simulink model "C6_Fix"  (R2024b)
settings: Solver=daessc  StartTime=0.0  StopTime=10.0  RelTol=1e-3  EnableMultiTasking=on
values from neighbouring files (symbols this model uses):
  Ix1 = 0.000555447536833    [C6_workspace.mat]
  Ix2 = 0.000647276077146    [C6_workspace.mat]
  Ix3 = 0.000647276077146    [C6_workspace.mat]
  Ix4 = 0.00061268668168    [C6_workspace.mat]
  Iy1 = 0.000281297083333    [C6_workspace.mat]
  Iy2 = 0.000285516539583    [C6_workspace.mat]
  Iy3 = 0.000285516539583    [C6_workspace.mat]
  Iy4 = 0.000286923025    [C6_workspace.mat]
  Iz1 = 0.000673203786833    [C6_workspace.mat]
  Iz2 = 0.000766798670896    [C6_workspace.mat]
  Iz3 = 0.000766798670896    [C6_workspace.mat]
  Iz4 = 0.00073279805668    [C6_workspace.mat]
  m_1 = 2    [C6_workspace.mat]
  m_2 = 2.03    [C6_workspace.mat]
  m_3 = 2.03    [C6_workspace.mat]
  m_4 = 2.04    [C6_workspace.mat]
undefined symbols (not defined in the file or in its folder): X, Y, Z
libraries: sm_lib x115, nesl_utility x25, robotcorelib x3, stm32f4xxblockslib x1
(part 1 of 6)
settings Model: STM32="{\"PWMOutput\":{\"ID\":\"C6_Fix:466\"}}"  ExtModeTrigDuration=2  Creator=steph  LastModifiedBy=steph
settings OptimizationCC: DefaultParameterBehavior=Inlined  EnhancedBackFolding=on  PassReuseOutputArgsAs=Individual arguments  ZeroExternalMemoryAtStartup=off  ZeroInternalMemoryAtStartup=off  MaxStackSize=512  OptimizeBlockOrder=speed  DifferentSizesBufferReuse=on  OptimizationCustomize=off  EfficientTunableParamExpr=on
settings DebuggingCC: ParameterTunabilityLossMsg=error
settings HardwareCC: ProdBitPerPointer=32  ProdBitPerSizeT=32  ProdBitPerPtrDiffT=32  ProdLargestAtomicInteger=Long  ProdLargestAtomicFloat=Double  ProdWordSize=32  ProdLongLongMode=on  ProdHWDeviceType=ARM Compatible->ARM Cortex-M
settings SFSimCC: MATLABDynamicMemAlloc=off
settings RTWCC: Description=Embedded Coder  SystemTargetFile=ert.tlc  HardwareBoard=STM32F4xx Based  TemplateMakefile=ert_default_tmf  Toolchain=GNU Tools for ARM Embedded Processors  BuildConfiguration=Faster Runs
settings CodeAppCC: ForceParamTrailComments=on  IgnoreCustomStorageClasses=off  OperatorAnnotations=on  SimulinkDataObjDesc=on  SFDataObjDesc=on  InsertBlockDesc=on
settings ERTTargetCC: TargetLangStandard=C99 (ISO)  CodeReplacementLibrary=ARM Cortex-M  RemoveResetFunc=off  ExtModeTransport=3  ExtModeStaticAlloc=on  ExtModeStaticAllocSize=2048  ExtModeMexFile=ext_xcp  ExtModeIntrfLevel=Level2 - Open  ConvertIfToSwitch=off  SuppressUnreachableDefaultCases=off

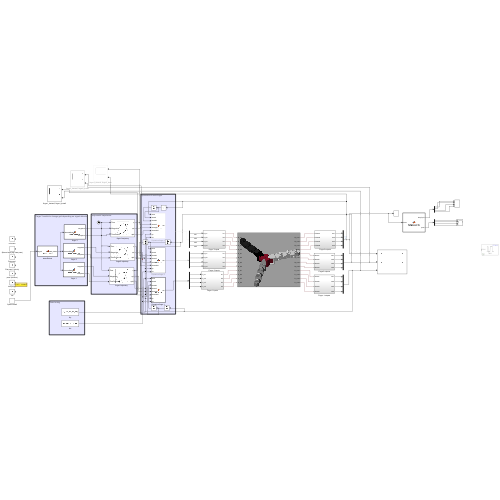
[thumbnail: Simulink's stored preview of the top-level diagram]
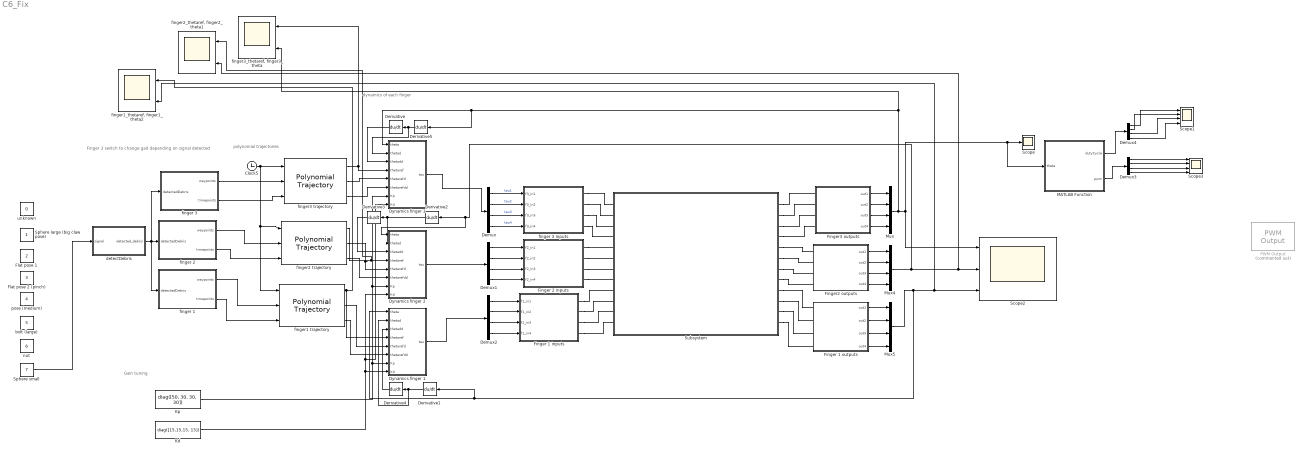
== system C6_Fix ==
  note: polynomial trajectories
  note: Gain tuning
  note: dynamics of each finger
  note: Finger 3 switch to change gait depending on signal detected
  Clock5 : Clock
  Demux{,1..4} (5 alike) : Demux
  Derivative{,1..5} (6 alike) : Derivative
  Dynamics finger 1 : MATLAB Function  TreatAsAtomicUnit=on
  Dynamics finger 2 : MATLAB Function  TreatAsAtomicUnit=on
  Dynamics finger 3 : MATLAB Function  TreatAsAtomicUnit=on
  Finger 1 inputs : Subsystem
  Finger 1 outputs : Subsystem
  Finger 2 inputs : Subsystem
  Finger2 outputs : Subsystem
  Finger3 outputs : Subsystem
  Flat pose 1 : Constant  Value=2
  Flat pose 2 (pinch) : Constant  Value=3
  Kd : Constant  Value=diag([15,15,15, 15])
  Kp : Constant  Value=diag([50, 30, 30, 30])
  MATLAB Function : MATLAB Function  TreatAsAtomicUnit=on
  Mux : Mux
  Mux4 : Mux
  Mux5 : Mux
  PWM Output : stm32f4xxblockslib/PWM Output  Commented=on  TimerModule=TIM1  DutycycleUnits=Percentage  EnableChannel1=on  EnableChannel2=off  EnableChannel3=off  EnableChannel4=off  EnableCounterInput=off  EnableMainOutputInput=off  EnableFrequencyInput=off  SetRCAfterCE=off  OutputDirection=off  OutputMainOutputEnableStatus=off  SampleTime=0.1  EnableSimPort=off  EnableUpdateEvent=off  EnableCaptureCompare1Event=off  EnableCaptureCompare2Event=off  EnableCaptureCompare3Event=off  EnableCaptureCompare4Event=off  EnableTriggerEvent=off  EnableBreakEvent=off  ProcessorFamily=STM32F4  hoistedMaskSrc=ECSoC/ECSimCodegen/PWM Output
  Scope : Scope
  Scope1 : Scope  NumInputPorts=4
  Scope2 : Scope  NumInputPorts=3
  Scope3 : Scope  NumInputPorts=4
  Sphere large (big claw pose) : Constant
  Sphere small : Constant  Value=7
  Subsystem : Subsystem
      mask Display: image('c6_fix.png');
  bolt (large) : Constant  Value=5
  detectDebris : MATLAB Function  TreatAsAtomicUnit=on
  finger 1 : MATLAB Function  TreatAsAtomicUnit=on
  finger 2 : MATLAB Function  TreatAsAtomicUnit=on
  finger 3 : MATLAB Function  TreatAsAtomicUnit=on
  finger 3 inputs : Subsystem
  finger1 trajectory : robotcorelib/Polynomial Trajectory  WaypointSource=External  Waypoints=[ 0, 2, 1, 5, 0; -1, 3, 1, 4, 4 ]  TimePoints=[ 0, 1, 2, 3, 4 ]  TimeInterval=[ 1, 4 ]  Method=Cubic Polynomial  ParameterSource=Internal  VelocityBoundaryCondition=zeros( 4, 10 )  AccelerationBoundaryCondition=zeros( 2, 5 )  SimulateUsing=Interpreted execution
  "finger1_thetaref, finger1_theta2" : Scope  NumInputPorts=2
  finger2 trajectory : robotcorelib/Polynomial Trajectory  WaypointSource=External  Waypoints=[ 0, 2, 1, 5, 0; -1, 3, 1, 4, 4 ]  TimePoints=[ 0, 1, 2, 3, 4 ]  TimeInterval=[ 1, 4 ]  Method=Cubic Polynomial  ParameterSource=Internal  VelocityBoundaryCondition=zeros( 4, 10 )  AccelerationBoundaryCondition=zeros( 2, 5 )  SimulateUsing=Interpreted execution
  "finger2_thetaref, finger2_theta1" : Scope  NumInputPorts=2
  finger3 trajectory : robotcorelib/Polynomial Trajectory  WaypointSource=External  Waypoints=[ 0, 2, 1, 5, 0; -1, 3, 1, 4, 4 ]  TimePoints=[ 0, 1, 2, 3, 4 ]  TimeInterval=[ 1, 4 ]  Method=Cubic Polynomial  ParameterSource=Internal  VelocityBoundaryCondition=zeros( 4, 10 )  AccelerationBoundaryCondition=zeros( 2, 5 )  SimulateUsing=Interpreted execution
  "finger3_thetaref, finger3_theta" : Scope  NumInputPorts=2
  nut : Constant  Value=6
  pose (medium) : Constant  Value=4
  unknown : Constant  Value=0
  wires:
  detectDebris/1(detected_debris) -> finger 1/1(detectedDebris), finger 2/1(detectedDebris), finger 3/1(detectedDebris)
  Finger2 outputs/1(out1) -> Mux4/1
  Demux1/3 -> Finger 2 inputs/3(f2_in3)
  finger1 trajectory/3 -> Dynamics finger 1/6(thetarefdd)
  Derivative2/1 -> Dynamics finger 2/2(thetad), Derivative3/1
  Finger3 outputs/4(out4) -> Mux/4
  Derivative3/1 -> Dynamics finger 2/3(thetadd)
  Finger2 outputs/4(out4) -> Mux4/4
  Demux2/3 -> Finger 1 inputs/3(f1_in3)
  finger3 trajectory/1 -> Dynamics finger 3/4(thetaref), "finger3_thetaref, finger3_theta"/1
  Demux/3 -> finger 3 inputs/3(f3_in3)  "tau3"
  finger 1/2(timepoints) -> finger1 trajectory/3
  Dynamics finger 1/1(tau) -> Demux2/1
  Derivative1/1 -> Dynamics finger 1/2(thetad), Derivative4/1
  Demux/2 -> finger 3 inputs/2(f3_in2)  "tau2"
  finger2 trajectory/3 -> Dynamics finger 2/6(thetarefdd)
  Derivative4/1 -> Dynamics finger 1/3(thetadd)
  Mux5/1 -> Dynamics finger 1/1(theta), Derivative1/1, "finger1_thetaref, finger1_theta2"/2, Scope2/3
  Demux1/4 -> Finger 2 inputs/4(f2_in4)
  Mux/1 -> "finger3_thetaref, finger3_theta"/2, Derivative5/1, Dynamics finger 3/1(theta), MATLAB Function/1(theta), Scope/1, Scope2/1
  Demux2/2 -> Finger 1 inputs/2(f1_in2)
  Derivative/1 -> Dynamics finger 3/3(thetadd)
  Finger3 outputs/3(out3) -> Mux/3
  finger1 trajectory/1 -> Dynamics finger 1/4(thetaref), "finger1_thetaref, finger1_theta2"/1
  finger3 trajectory/2 -> Dynamics finger 3/5(thetarefd)
  Finger 1 outputs/3(out3) -> Mux5/3
  Clock5/1 -> finger3 trajectory/1, finger2 trajectory/1, finger1 trajectory/1
  Kp/1 -> Dynamics finger 1/7(Kp), Dynamics finger 2/7(Kp), Dynamics finger 3/7(Kp)
  finger 1/1(waypoints) -> finger1 trajectory/2
  Demux1/1 -> Finger 2 inputs/1(f2_in1)
  Demux2/4 -> Finger 1 inputs/4(f1_in4)
  Demux2/1 -> Finger 1 inputs/1(f1_in1)
  Dynamics finger 3/1(tau) -> Demux/1
  Finger 1 outputs/2(out2) -> Mux5/2
  Mux4/1 -> Dynamics finger 2/1(theta), Derivative2/1, "finger2_thetaref, finger2_theta1"/2, Scope2/2
  finger2 trajectory/2 -> Dynamics finger 2/5(thetarefd)
  Demux1/2 -> Finger 2 inputs/2(f2_in2)
  finger2 trajectory/1 -> "finger2_thetaref, finger2_theta1"/1, Dynamics finger 2/4(thetaref)
  finger 2/2(timepoints) -> finger2 trajectory/3
  Finger2 outputs/2(out2) -> Mux4/2
  Finger 1 outputs/1(out1) -> Mux5/1
  finger3 trajectory/3 -> Dynamics finger 3/6(thetarefdd)
  Demux/4 -> finger 3 inputs/4(f3_in4)  "tau4"
  finger 3/1(waypoints) -> finger3 trajectory/2
  finger 3/2(timepoints) -> finger3 trajectory/3
  finger1 trajectory/2 -> Dynamics finger 1/5(thetarefd)
  Dynamics finger 2/1(tau) -> Demux1/1
  finger 2/1(waypoints) -> finger2 trajectory/2
  Kd/1 -> Dynamics finger 1/8(Kd), Dynamics finger 2/8(Kd), Dynamics finger 3/8(Kd)
  Demux/1 -> finger 3 inputs/1(f3_in1)  "tau1"
  Finger3 outputs/1(out1) -> Mux/1
  Finger2 outputs/3(out3) -> Mux4/3
  Finger 1 outputs/4(out4) -> Mux5/4
  Finger3 outputs/2(out2) -> Mux/2
  Derivative5/1 -> Dynamics finger 3/2(thetad), Derivative/1
  MATLAB Function/2(pwm) -> Demux3/1
  Demux3/1 -> Scope3/1
  Demux3/2 -> Scope3/2
  Demux3/3 -> Scope3/3
  Demux3/4 -> Scope3/4
  MATLAB Function/1(dutyCycle) -> Demux4/1
  Demux4/1 -> Scope1/1
  Demux4/2 -> Scope1/2
  Demux4/3 -> Scope1/3
  Demux4/4 -> Scope1/4
  Sphere small/1 -> detectDebris/1(signal)
  connections:
  Subsystem/RConn2 -- Finger3 outputs/LConn2
  Finger 1 inputs/RConn2 -- Subsystem/LConn10
  Subsystem/RConn5 -- Finger2 outputs/LConn1
  finger 3 inputs/RConn2 -- Subsystem/LConn2
  Finger 1 inputs/RConn4 -- Subsystem/LConn12
  Subsystem/RConn8 -- Finger2 outputs/LConn4
  finger 3 inputs/RConn4 -- Subsystem/LConn4
  Subsystem/RConn11 -- Finger 1 outputs/LConn3
  finger 3 inputs/RConn3 -- Subsystem/LConn3
  Finger 2 inputs/RConn4 -- Subsystem/LConn8
  Subsystem/RConn4 -- Finger3 outputs/LConn4
  Finger 1 inputs/RConn1 -- Subsystem/LConn9
  Subsystem/RConn10 -- Finger 1 outputs/LConn2
  Finger 2 inputs/RConn1 -- Subsystem/LConn5
  Subsystem/RConn3 -- Finger3 outputs/LConn3
  Finger 2 inputs/RConn2 -- Subsystem/LConn6
  Subsystem/RConn7 -- Finger2 outputs/LConn3
  finger 3 inputs/RConn1 -- Subsystem/LConn1
  Finger 2 inputs/RConn3 -- Subsystem/LConn7
  Subsystem/RConn12 -- Finger 1 outputs/LConn4
  Finger 1 inputs/RConn3 -- Subsystem/LConn11
  Subsystem/RConn9 -- Finger 1 outputs/LConn1
  Subsystem/RConn1 -- Finger3 outputs/LConn1
  Subsystem/RConn6 -- Finger2 outputs/LConn2

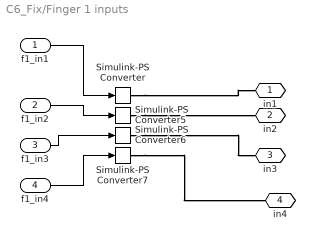
== system C6_Fix/Finger 1 inputs ==
  f1_in1 : Inport
  f1_in2 : Inport  Port=2
  f1_in3 : Inport  Port=3
  f1_in4 : Inport  Port=4
  Simulink-PS Converter{,5..7} (4 alike) : nesl_utility/Simulink-PS Converter  PhysicalDomain=network_engine_domain  SubClassName=ps_input  LeftPortType=input  RightPortType=output  PseudoPeriodic=off  Frequencies=[]  NoiseDistribution=none  NoiseParameters=[]  Unit=1  AffineConversion=off  FilteringAndDerivatives=provide  SimscapeFilterOrder=1  InputFilterTimeConstant=0.001  UdotUserProvided=0
  in1 : PMIOPort  Side=Right
  in2 : PMIOPort  Port=2  Side=Right
  in3 : PMIOPort  Port=3  Side=Right
  in4 : PMIOPort  Port=4  Side=Right
  wires:
  f1_in2/1 -> Simulink-PS Converter5/1
  f1_in4/1 -> Simulink-PS Converter7/1
  f1_in1/1 -> Simulink-PS Converter/1
  f1_in3/1 -> Simulink-PS Converter6/1
  connections:
  Simulink-PS Converter5/RConn1 -- in2/RConn1
  Simulink-PS Converter7/RConn1 -- in4/RConn1
  Simulink-PS Converter6/RConn1 -- in3/RConn1
  Simulink-PS Converter/RConn1 -- in1/RConn1

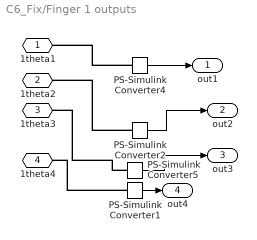
== system C6_Fix/Finger 1 outputs ==
  PS-Simulink Converter{1..2,4..5} (4 alike) : nesl_utility/PS-Simulink Converter  PhysicalDomain=network_engine_domain  SubClassName=ps_output  LeftPortType=input  RightPortType=output  PseudoPeriodic=off  Frequencies=[]  VectorFormat=inherit  Unit=inherit  AffineConversion=off
  1theta1 : PMIOPort  Side=Left
  1theta2 : PMIOPort  Port=2  Side=Left
  1theta3 : PMIOPort  Port=3  Side=Left
  1theta4 : PMIOPort  Port=4  Side=Left
  out1 : Outport
  out2 : Outport  Port=2
  out3 : Outport  Port=3
  out4 : Outport  Port=4
  wires:
  PS-Simulink Converter5/1 -> out3/1
  PS-Simulink Converter1/1 -> out4/1
  PS-Simulink Converter4/1 -> out1/1
  PS-Simulink Converter2/1 -> out2/1
  connections:
  PS-Simulink Converter2/LConn1 -- 1theta2/RConn1
  PS-Simulink Converter1/LConn1 -- 1theta4/RConn1
  PS-Simulink Converter4/LConn1 -- 1theta1/RConn1
  PS-Simulink Converter5/LConn1 -- 1theta3/RConn1

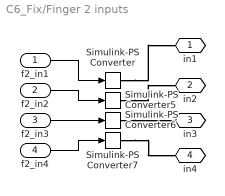
== system C6_Fix/Finger 2 inputs ==
  f2_in1 : Inport
  f2_in2 : Inport  Port=2
  f2_in3 : Inport  Port=3
  f2_in4 : Inport  Port=4
  Simulink-PS Converter{,5..7} (4 alike) : nesl_utility/Simulink-PS Converter  PhysicalDomain=network_engine_domain  SubClassName=ps_input  LeftPortType=input  RightPortType=output  PseudoPeriodic=off  Frequencies=[]  NoiseDistribution=none  NoiseParameters=[]  Unit=1  AffineConversion=off  FilteringAndDerivatives=provide  SimscapeFilterOrder=1  InputFilterTimeConstant=0.001  UdotUserProvided=0
  in1 : PMIOPort  Side=Right
  in2 : PMIOPort  Port=2  Side=Right
  in3 : PMIOPort  Port=3  Side=Right
  in4 : PMIOPort  Port=4  Side=Right
  wires:
  f2_in3/1 -> Simulink-PS Converter6/1
  f2_in2/1 -> Simulink-PS Converter5/1
  f2_in4/1 -> Simulink-PS Converter7/1
  f2_in1/1 -> Simulink-PS Converter/1
  connections:
  Simulink-PS Converter7/RConn1 -- in4/RConn1
  Simulink-PS Converter5/RConn1 -- in2/RConn1
  Simulink-PS Converter6/RConn1 -- in3/RConn1
  Simulink-PS Converter/RConn1 -- in1/RConn1

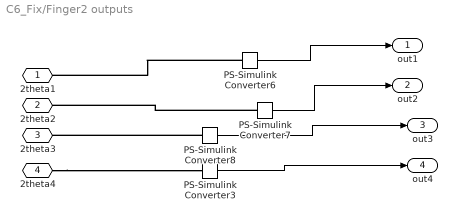
== system C6_Fix/Finger2 outputs ==
  PS-Simulink Converter{3,6..8} (4 alike) : nesl_utility/PS-Simulink Converter  PhysicalDomain=network_engine_domain  SubClassName=ps_output  LeftPortType=input  RightPortType=output  PseudoPeriodic=off  Frequencies=[]  VectorFormat=inherit  Unit=inherit  AffineConversion=off
  2theta1 : PMIOPort  Side=Left
  2theta2 : PMIOPort  Port=2  Side=Left
  2theta3 : PMIOPort  Port=3  Side=Left
  2theta4 : PMIOPort  Port=4  Side=Left
  out1 : Outport
  out2 : Outport  Port=2
  out3 : Outport  Port=3
  out4 : Outport  Port=4
  wires:
  PS-Simulink Converter6/1 -> out1/1
  PS-Simulink Converter3/1 -> out4/1
  PS-Simulink Converter7/1 -> out2/1
  PS-Simulink Converter8/1 -> out3/1
  connections:
  2theta4/RConn1 -- PS-Simulink Converter3/LConn1
  PS-Simulink Converter7/LConn1 -- 2theta2/RConn1
  PS-Simulink Converter6/LConn1 -- 2theta1/RConn1
  PS-Simulink Converter8/LConn1 -- 2theta3/RConn1

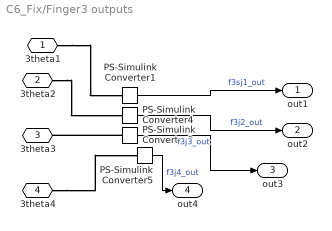
== system C6_Fix/Finger3 outputs ==
  PS-Simulink Converter{1..2,4..5} (4 alike) : nesl_utility/PS-Simulink Converter  PhysicalDomain=network_engine_domain  SubClassName=ps_output  LeftPortType=input  RightPortType=output  PseudoPeriodic=off  Frequencies=[]  VectorFormat=inherit  Unit=inherit  AffineConversion=off
  3theta1 : PMIOPort  Side=Left
  3theta2 : PMIOPort  Port=2  Side=Left
  3theta3 : PMIOPort  Port=3  Side=Left
  3theta4 : PMIOPort  Port=4  Side=Left
  out1 : Outport
  out2 : Outport  Port=2
  out3 : Outport  Port=3
  out4 : Outport  Port=4
  wires:
  PS-Simulink Converter4/1 -> out2/1  "f3j2_out"
  PS-Simulink Converter1/1 -> out1/1  "f3sj1_out"
  PS-Simulink Converter2/1 -> out3/1  "f3j3_out"
  PS-Simulink Converter5/1 -> out4/1  "f3j4_out"
  connections:
  PS-Simulink Converter2/LConn1 -- 3theta3/RConn1
  3theta1/RConn1 -- PS-Simulink Converter1/LConn1
  3theta2/RConn1 -- PS-Simulink Converter4/LConn1
  3theta4/RConn1 -- PS-Simulink Converter5/LConn1

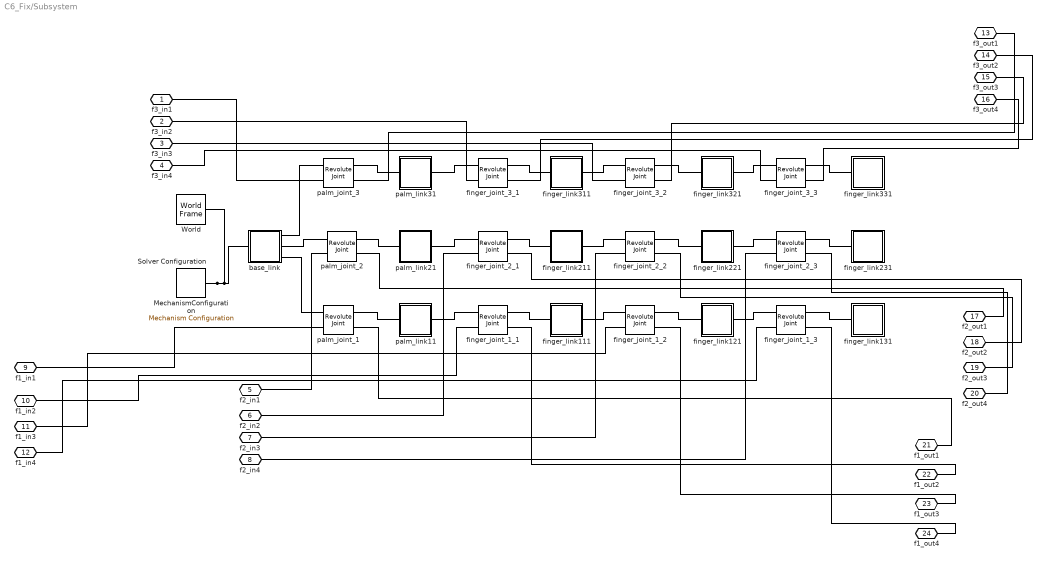
== system C6_Fix/Subsystem ==
  MechanismConfiguration : sm_lib/Utilities/Mechanism Configuration  UniformGravity=Constant  GravityVector=[0 0 -9.80665]  GravityVectorUnits=m/s^2  LinearizationDelta=0.001  JointModeTransitionNonlinearIterations=2
  Solver Configuration : nesl_utility/Solver Configuration  PhysicalDomain=network_engine_domain  SubClassName=solver  LeftPortType=input  RightPortType=generic  Tones=[]  Harmonics=[]  SimulateNoise=off  Profile=off  UseLocalSampling=off  EnableSwitchedLinearOptims=on  FrequencyDomain=off  UseCCode=off  RelTol=0.001  AbsTol=0.001  MinStep=1e-09  ToWorkspace=off  RevertToSquareIcSolve=off  NumHomotopyIterations=100  PhasorMode=off  PhasorModeNumHarmonics=1  ConsistencySolver=NEWTON_XTOL_AFTER_FTOL  IndexReductionMethod=DerivativeReplacement  DoDC=off  ResidualTolerance=1e-09  ConsistencyTolSource=GLOBAL  ConsistencyAbsTol=0.001  ConsistencyRelTol=0.001  ConsistencyTolFactor=0.001  UseLocalSolver=off  LocalSolverChoice=NE_BACKWARD_EULER_ADVANCER  ResolveIndetEquations=on  FunctionEvalNumThread=1  LocalSolverSampleTime=0.001  DoFixedCost=off  MaxNonlinIter=3  MaxModeIter=2  ComputeImpulses=off  ImpulseIterations=2  LinearAlgebra=auto  LinearAlgebraNumThread=0  EquationFormulation=NE_TIME_EF  DelaysMemoryBudget=1024  AutomaticFiltering=on  FilteringTimeConstant=0.001  PartitionStorageMethod=AS_NEEDED  PartitionMemoryBudget=1024  PartitionMethod=ROBUST  MultibodyUseLocalSolver=off  MultibodyLocalSolverChoice=ODE1  MultibodyLocalSolverSampleTime=0.001
  World : sm_lib/Frames and Transforms/World Frame
  base_link : Subsystem
  finger_joint_1_1 : sm_lib/Joints/Revolute Joint  JointMode=Normal  CompositeWrenchDir=FollowerOnBase  CompositeWrenchFrame=BaseFrame  SenseConstraintForce=off  SenseConstraintTorque=off  SenseTotalForce=off  SenseTotalTorque=off  PositionTargetSpecify=off  PositionTargetPriority=High  PositionTargetValue=0  PositionTargetValueUnits=deg  VelocityTargetSpecify=off  VelocityTargetPriority=High  VelocityTargetValue=0  VelocityTargetValueUnits=deg/s  EquilibriumPosition=0  EquilibriumPositionUnits=deg  SpringStiffness=0  SpringStiffnessUnits=N*m/deg  DampingCoefficient=0  DampingCoefficientUnits=kg*m^2/(rad*s)  LowerLimitSpecify=on  LowerLimitBound=0  LowerLimitBoundUnits=rad  LowerLimitStiffness=1e4  LowerLimitStiffnessUnits=N*m/deg  LowerLimitDamping=10  LowerLimitDampingUnits=N*m/(deg/s)  LowerLimitTransitionRegionWidth=0.1  LowerLimitTransitionRegionWidthUnits=deg  UpperLimitSpecify=on  UpperLimitBound=1.570796  UpperLimitBoundUnits=rad  UpperLimitStiffness=1e4  UpperLimitStiffnessUnits=N*m/deg  UpperLimitDamping=10  UpperLimitDampingUnits=N*m/(deg/s)  UpperLimitTransitionRegionWidth=0.1  UpperLimitTransitionRegionWidthUnits=deg  TorqueActuationMode=InputTorque  MotionActuationMode=ComputedMotion  SensePosition=on  SenseVelocity=off  SenseAcceleration=off  SenseTorqueForce=off  SenseLowerLimitTorqueForce=off  SenseUpperLimitTorqueForce=off
  finger_joint_1_2 : sm_lib/Joints/Revolute Joint  JointMode=Normal  CompositeWrenchDir=FollowerOnBase  CompositeWrenchFrame=BaseFrame  SenseConstraintForce=off  SenseConstraintTorque=off  SenseTotalForce=off  SenseTotalTorque=off  PositionTargetSpecify=off  PositionTargetPriority=High  PositionTargetValue=0  PositionTargetValueUnits=deg  VelocityTargetSpecify=off  VelocityTargetPriority=High  VelocityTargetValue=0  VelocityTargetValueUnits=deg/s  EquilibriumPosition=0  EquilibriumPositionUnits=deg  SpringStiffness=0  SpringStiffnessUnits=N*m/deg  DampingCoefficient=0  DampingCoefficientUnits=kg*m^2/(rad*s)  LowerLimitSpecify=on  LowerLimitBound=0  LowerLimitBoundUnits=rad  LowerLimitStiffness=1e4  LowerLimitStiffnessUnits=N*m/deg  LowerLimitDamping=10  LowerLimitDampingUnits=N*m/(deg/s)  LowerLimitTransitionRegionWidth=0.1  LowerLimitTransitionRegionWidthUnits=deg  UpperLimitSpecify=on  UpperLimitBound=1.570796  UpperLimitBoundUnits=rad  UpperLimitStiffness=1e4  UpperLimitStiffnessUnits=N*m/deg  UpperLimitDamping=10  UpperLimitDampingUnits=N*m/(deg/s)  UpperLimitTransitionRegionWidth=0.1  UpperLimitTransitionRegionWidthUnits=deg  TorqueActuationMode=InputTorque  MotionActuationMode=ComputedMotion  SensePosition=on  SenseVelocity=off  SenseAcceleration=off  SenseTorqueForce=off  SenseLowerLimitTorqueForce=off  SenseUpperLimitTorqueForce=off
  finger_joint_1_3 : sm_lib/Joints/Revolute Joint  JointMode=Normal  CompositeWrenchDir=FollowerOnBase  CompositeWrenchFrame=BaseFrame  SenseConstraintForce=off  SenseConstraintTorque=off  SenseTotalForce=off  SenseTotalTorque=off  PositionTargetSpecify=off  PositionTargetPriority=High  PositionTargetValue=0  PositionTargetValueUnits=deg  VelocityTargetSpecify=off  VelocityTargetPriority=High  VelocityTargetValue=0  VelocityTargetValueUnits=deg/s  EquilibriumPosition=0  EquilibriumPositionUnits=deg  SpringStiffness=0  SpringStiffnessUnits=N*m/deg  DampingCoefficient=0  DampingCoefficientUnits=kg*m^2/(rad*s)  LowerLimitSpecify=on  LowerLimitBound=-pi/2  LowerLimitBoundUnits=rad  LowerLimitStiffness=1e4  LowerLimitStiffnessUnits=N*m/deg  LowerLimitDamping=10  LowerLimitDampingUnits=N*m/(deg/s)  LowerLimitTransitionRegionWidth=0.1  LowerLimitTransitionRegionWidthUnits=deg  UpperLimitSpecify=on  UpperLimitBound=pi/2  UpperLimitBoundUnits=rad  UpperLimitStiffness=1e4  UpperLimitStiffnessUnits=N*m/deg  UpperLimitDamping=10  UpperLimitDampingUnits=N*m/(deg/s)  UpperLimitTransitionRegionWidth=0.1  UpperLimitTransitionRegionWidthUnits=deg  TorqueActuationMode=InputTorque  MotionActuationMode=ComputedMotion  SensePosition=on  SenseVelocity=off  SenseAcceleration=off  SenseTorqueForce=off  SenseLowerLimitTorqueForce=off  SenseUpperLimitTorqueForce=off
  finger_joint_2_1 : sm_lib/Joints/Revolute Joint  JointMode=Normal  CompositeWrenchDir=FollowerOnBase  CompositeWrenchFrame=BaseFrame  SenseConstraintForce=off  SenseConstraintTorque=off  SenseTotalForce=off  SenseTotalTorque=off  PositionTargetSpecify=off  PositionTargetPriority=High  PositionTargetValue=0  PositionTargetValueUnits=deg  VelocityTargetSpecify=off  VelocityTargetPriority=High  VelocityTargetValue=0  VelocityTargetValueUnits=deg/s  EquilibriumPosition=0  EquilibriumPositionUnits=deg  SpringStiffness=0  SpringStiffnessUnits=N*m/deg  DampingCoefficient=0  DampingCoefficientUnits=kg*m^2/(rad*s)  LowerLimitSpecify=on  LowerLimitBound=0  LowerLimitBoundUnits=rad  LowerLimitStiffness=1e4  LowerLimitStiffnessUnits=N*m/deg  LowerLimitDamping=10  LowerLimitDampingUnits=N*m/(deg/s)  LowerLimitTransitionRegionWidth=0.1  LowerLimitTransitionRegionWidthUnits=deg  UpperLimitSpecify=on  UpperLimitBound=1.570796  UpperLimitBoundUnits=rad  UpperLimitStiffness=1e4  UpperLimitStiffnessUnits=N*m/deg  UpperLimitDamping=10  UpperLimitDampingUnits=N*m/(deg/s)  UpperLimitTransitionRegionWidth=0.1  UpperLimitTransitionRegionWidthUnits=deg  TorqueActuationMode=InputTorque  MotionActuationMode=ComputedMotion  SensePosition=on  SenseVelocity=off  SenseAcceleration=off  SenseTorqueForce=off  SenseLowerLimitTorqueForce=off  SenseUpperLimitTorqueForce=off
  finger_joint_2_2 : sm_lib/Joints/Revolute Joint  JointMode=Normal  CompositeWrenchDir=FollowerOnBase  CompositeWrenchFrame=BaseFrame  SenseConstraintForce=off  SenseConstraintTorque=off  SenseTotalForce=off  SenseTotalTorque=off  PositionTargetSpecify=off  PositionTargetPriority=High  PositionTargetValue=0  PositionTargetValueUnits=deg  VelocityTargetSpecify=off  VelocityTargetPriority=High  VelocityTargetValue=0  VelocityTargetValueUnits=deg/s  EquilibriumPosition=0  EquilibriumPositionUnits=deg  SpringStiffness=0  SpringStiffnessUnits=N*m/deg  DampingCoefficient=0  DampingCoefficientUnits=kg*m^2/(rad*s)  LowerLimitSpecify=on  LowerLimitBound=0  LowerLimitBoundUnits=rad  LowerLimitStiffness=1e4  LowerLimitStiffnessUnits=N*m/deg  LowerLimitDamping=10  LowerLimitDampingUnits=N*m/(deg/s)  LowerLimitTransitionRegionWidth=0.1  LowerLimitTransitionRegionWidthUnits=deg  UpperLimitSpecify=on  UpperLimitBound=1.570796  UpperLimitBoundUnits=rad  UpperLimitStiffness=1e4  UpperLimitStiffnessUnits=N*m/deg  UpperLimitDamping=10  UpperLimitDampingUnits=N*m/(deg/s)  UpperLimitTransitionRegionWidth=0.1  UpperLimitTransitionRegionWidthUnits=deg  TorqueActuationMode=InputTorque  MotionActuationMode=ComputedMotion  SensePosition=on  SenseVelocity=off  SenseAcceleration=off  SenseTorqueForce=off  SenseLowerLimitTorqueForce=off  SenseUpperLimitTorqueForce=off
  finger_joint_2_3 : sm_lib/Joints/Revolute Joint  JointMode=Normal  CompositeWrenchDir=FollowerOnBase  CompositeWrenchFrame=BaseFrame  SenseConstraintForce=off  SenseConstraintTorque=off  SenseTotalForce=off  SenseTotalTorque=off  PositionTargetSpecify=off  PositionTargetPriority=High  PositionTargetValue=0  PositionTargetValueUnits=deg  VelocityTargetSpecify=off  VelocityTargetPriority=High  VelocityTargetValue=0  VelocityTargetValueUnits=deg/s  EquilibriumPosition=0  EquilibriumPositionUnits=deg  SpringStiffness=0  SpringStiffnessUnits=N*m/deg  DampingCoefficient=0  DampingCoefficientUnits=kg*m^2/(rad*s)  LowerLimitSpecify=on  LowerLimitBound=-pi/2  LowerLimitBoundUnits=rad  LowerLimitStiffness=1e4  LowerLimitStiffnessUnits=N*m/deg  LowerLimitDamping=10  LowerLimitDampingUnits=N*m/(deg/s)  LowerLimitTransitionRegionWidth=0.1  LowerLimitTransitionRegionWidthUnits=deg  UpperLimitSpecify=on  UpperLimitBound=pi/2  UpperLimitBoundUnits=rad  UpperLimitStiffness=1e4  UpperLimitStiffnessUnits=N*m/deg  UpperLimitDamping=10  UpperLimitDampingUnits=N*m/(deg/s)  UpperLimitTransitionRegionWidth=0.1  UpperLimitTransitionRegionWidthUnits=deg  TorqueActuationMode=InputTorque  MotionActuationMode=ComputedMotion  SensePosition=on  SenseVelocity=off  SenseAcceleration=off  SenseTorqueForce=off  SenseLowerLimitTorqueForce=off  SenseUpperLimitTorqueForce=off
  finger_joint_3_1 : sm_lib/Joints/Revolute Joint  JointMode=Normal  CompositeWrenchDir=FollowerOnBase  CompositeWrenchFrame=BaseFrame  SenseConstraintForce=off  SenseConstraintTorque=off  SenseTotalForce=off  SenseTotalTorque=off  PositionTargetSpecify=off  PositionTargetPriority=High  PositionTargetValue=0  PositionTargetValueUnits=deg  VelocityTargetSpecify=off  VelocityTargetPriority=High  VelocityTargetValue=0  VelocityTargetValueUnits=deg/s  EquilibriumPosition=0  EquilibriumPositionUnits=deg  SpringStiffness=0  SpringStiffnessUnits=N*m/deg  DampingCoefficient=0  DampingCoefficientUnits=kg*m^2/(rad*s)  LowerLimitSpecify=on  LowerLimitBound=0  LowerLimitBoundUnits=rad  LowerLimitStiffness=1e4  LowerLimitStiffnessUnits=N*m/deg  LowerLimitDamping=10  LowerLimitDampingUnits=N*m/(deg/s)  LowerLimitTransitionRegionWidth=0.1  LowerLimitTransitionRegionWidthUnits=deg  UpperLimitSpecify=on  UpperLimitBound=1.570796  UpperLimitBoundUnits=rad  UpperLimitStiffness=1e4  UpperLimitStiffnessUnits=N*m/deg  UpperLimitDamping=10  UpperLimitDampingUnits=N*m/(deg/s)  UpperLimitTransitionRegionWidth=0.1  UpperLimitTransitionRegionWidthUnits=deg  TorqueActuationMode=InputTorque  MotionActuationMode=ComputedMotion  SensePosition=on  SenseVelocity=off  SenseAcceleration=off  SenseTorqueForce=off  SenseLowerLimitTorqueForce=off  SenseUpperLimitTorqueForce=off
  finger_joint_3_2 : sm_lib/Joints/Revolute Joint  JointMode=Normal  CompositeWrenchDir=FollowerOnBase  CompositeWrenchFrame=BaseFrame  SenseConstraintForce=off  SenseConstraintTorque=off  SenseTotalForce=off  SenseTotalTorque=off  PositionTargetSpecify=off  PositionTargetPriority=High  PositionTargetValue=0  PositionTargetValueUnits=deg  VelocityTargetSpecify=off  VelocityTargetPriority=High  VelocityTargetValue=0  VelocityTargetValueUnits=deg/s  EquilibriumPosition=0  EquilibriumPositionUnits=deg  SpringStiffness=0  SpringStiffnessUnits=N*m/deg  DampingCoefficient=0  DampingCoefficientUnits=kg*m^2/(rad*s)  LowerLimitSpecify=on  LowerLimitBound=0  LowerLimitBoundUnits=rad  LowerLimitStiffness=1e4  LowerLimitStiffnessUnits=N*m/deg  LowerLimitDamping=10  LowerLimitDampingUnits=N*m/(deg/s)  LowerLimitTransitionRegionWidth=0.1  LowerLimitTransitionRegionWidthUnits=deg  UpperLimitSpecify=on  UpperLimitBound=1.570796  UpperLimitBoundUnits=rad  UpperLimitStiffness=1e4  UpperLimitStiffnessUnits=N*m/deg  UpperLimitDamping=10  UpperLimitDampingUnits=N*m/(deg/s)  UpperLimitTransitionRegionWidth=0.1  UpperLimitTransitionRegionWidthUnits=deg  TorqueActuationMode=InputTorque  MotionActuationMode=ComputedMotion  SensePosition=on  SenseVelocity=off  SenseAcceleration=off  SenseTorqueForce=off  SenseLowerLimitTorqueForce=off  SenseUpperLimitTorqueForce=off
  finger_joint_3_3 : sm_lib/Joints/Revolute Joint  JointMode=Normal  CompositeWrenchDir=FollowerOnBase  CompositeWrenchFrame=BaseFrame  SenseConstraintForce=off  SenseConstraintTorque=off  SenseTotalForce=off  SenseTotalTorque=off  PositionTargetSpecify=off  PositionTargetPriority=High  PositionTargetValue=0  PositionTargetValueUnits=deg  VelocityTargetSpecify=off  VelocityTargetPriority=High  VelocityTargetValue=0  VelocityTargetValueUnits=deg/s  EquilibriumPosition=0  EquilibriumPositionUnits=deg  SpringStiffness=0  SpringStiffnessUnits=N*m/deg  DampingCoefficient=0  DampingCoefficientUnits=kg*m^2/(rad*s)  LowerLimitSpecify=on  LowerLimitBound=-pi/2  LowerLimitBoundUnits=rad  LowerLimitStiffness=1e4  LowerLimitStiffnessUnits=N*m/deg  LowerLimitDamping=10  LowerLimitDampingUnits=N*m/(deg/s)  LowerLimitTransitionRegionWidth=0.1  LowerLimitTransitionRegionWidthUnits=deg  UpperLimitSpecify=on  UpperLimitBound=pi/2  UpperLimitBoundUnits=rad  UpperLimitStiffness=1e4  UpperLimitStiffnessUnits=N*m/deg  UpperLimitDamping=10  UpperLimitDampingUnits=N*m/(deg/s)  UpperLimitTransitionRegionWidth=0.1  UpperLimitTransitionRegionWidthUnits=deg  TorqueActuationMode=InputTorque  MotionActuationMode=ComputedMotion  SensePosition=on  SenseVelocity=off  SenseAcceleration=off  SenseTorqueForce=off  SenseLowerLimitTorqueForce=off  SenseUpperLimitTorqueForce=off
  finger_link111 : Subsystem
  finger_link121 : Subsystem
  finger_link131 : Subsystem
  finger_link211 : Subsystem
  finger_link221 : Subsystem
  finger_link231 : Subsystem
  finger_link311 : Subsystem
  finger_link321 : Subsystem
  finger_link331 : Subsystem
  palm_joint_1 : sm_lib/Joints/Revolute Joint  JointMode=Normal  CompositeWrenchDir=FollowerOnBase  CompositeWrenchFrame=BaseFrame  SenseConstraintForce=off  SenseConstraintTorque=off  SenseTotalForce=off  SenseTotalTorque=off  PositionTargetSpecify=off  PositionTargetPriority=High  PositionTargetValue=0  PositionTargetValueUnits=deg  VelocityTargetSpecify=off  VelocityTargetPriority=High  VelocityTargetValue=0  VelocityTargetValueUnits=deg/s  EquilibriumPosition=0  EquilibriumPositionUnits=deg  SpringStiffness=0  SpringStiffnessUnits=N*m/deg  DampingCoefficient=0  DampingCoefficientUnits=kg*m^2/(rad*s)  LowerLimitSpecify=on  LowerLimitBound=-0.523599  LowerLimitBoundUnits=rad  LowerLimitStiffness=1e4  LowerLimitStiffnessUnits=N*m/deg  LowerLimitDamping=10  LowerLimitDampingUnits=N*m/(deg/s)  LowerLimitTransitionRegionWidth=0.1  LowerLimitTransitionRegionWidthUnits=deg  UpperLimitSpecify=on  UpperLimitBound=0.523599  UpperLimitBoundUnits=rad  UpperLimitStiffness=1e4  UpperLimitStiffnessUnits=N*m/deg  UpperLimitDamping=10  UpperLimitDampingUnits=N*m/(deg/s)  UpperLimitTransitionRegionWidth=0.1  UpperLimitTransitionRegionWidthUnits=deg  TorqueActuationMode=InputTorque  MotionActuationMode=ComputedMotion  SensePosition=on  SenseVelocity=off  SenseAcceleration=off  SenseTorqueForce=off  SenseLowerLimitTorqueForce=off  SenseUpperLimitTorqueForce=off
  palm_joint_2 : sm_lib/Joints/Revolute Joint  JointMode=Normal  CompositeWrenchDir=FollowerOnBase  CompositeWrenchFrame=BaseFrame  SenseConstraintForce=off  SenseConstraintTorque=off  SenseTotalForce=off  SenseTotalTorque=off  PositionTargetSpecify=off  PositionTargetPriority=High  PositionTargetValue=0  PositionTargetValueUnits=deg  VelocityTargetSpecify=off  VelocityTargetPriority=High  VelocityTargetValue=0  VelocityTargetValueUnits=deg/s  EquilibriumPosition=0  EquilibriumPositionUnits=deg  SpringStiffness=0  SpringStiffnessUnits=N*m/deg  DampingCoefficient=0  DampingCoefficientUnits=kg*m^2/(rad*s)  LowerLimitSpecify=on  LowerLimitBound=-0.523599  LowerLimitBoundUnits=rad  LowerLimitStiffness=1e4  LowerLimitStiffnessUnits=N*m/deg  LowerLimitDamping=10  LowerLimitDampingUnits=N*m/(deg/s)  LowerLimitTransitionRegionWidth=0.1  LowerLimitTransitionRegionWidthUnits=deg  UpperLimitSpecify=on  UpperLimitBound=0.523599  UpperLimitBoundUnits=rad  UpperLimitStiffness=1e4  UpperLimitStiffnessUnits=N*m/deg  UpperLimitDamping=10  UpperLimitDampingUnits=N*m/(deg/s)  UpperLimitTransitionRegionWidth=0.1  UpperLimitTransitionRegionWidthUnits=deg  TorqueActuationMode=InputTorque  MotionActuationMode=ComputedMotion  SensePosition=on  SenseVelocity=off  SenseAcceleration=off  SenseTorqueForce=off  SenseLowerLimitTorqueForce=off  SenseUpperLimitTorqueForce=off
  palm_joint_3 : sm_lib/Joints/Revolute Joint  JointMode=Normal  CompositeWrenchDir=FollowerOnBase  CompositeWrenchFrame=BaseFrame  SenseConstraintForce=off  SenseConstraintTorque=off  SenseTotalForce=off  SenseTotalTorque=off  PositionTargetSpecify=off  PositionTargetPriority=High  PositionTargetValue=0  PositionTargetValueUnits=deg  VelocityTargetSpecify=off  VelocityTargetPriority=High  VelocityTargetValue=0  VelocityTargetValueUnits=deg/s  EquilibriumPosition=0  EquilibriumPositionUnits=deg  SpringStiffness=0  SpringStiffnessUnits=N*m/deg  DampingCoefficient=0  DampingCoefficientUnits=kg*m^2/(rad*s)  LowerLimitSpecify=on  LowerLimitBound=-0.523599  LowerLimitBoundUnits=rad  LowerLimitStiffness=1e4  LowerLimitStiffnessUnits=N*m/deg  LowerLimitDamping=10  LowerLimitDampingUnits=N*m/(deg/s)  LowerLimitTransitionRegionWidth=0.1  LowerLimitTransitionRegionWidthUnits=deg  UpperLimitSpecify=on  UpperLimitBound=0.523599  UpperLimitBoundUnits=rad  UpperLimitStiffness=1e4  UpperLimitStiffnessUnits=N*m/deg  UpperLimitDamping=10  UpperLimitDampingUnits=N*m/(deg/s)  UpperLimitTransitionRegionWidth=0.1  UpperLimitTransitionRegionWidthUnits=deg  TorqueActuationMode=InputTorque  MotionActuationMode=ComputedMotion  SensePosition=on  SenseVelocity=off  SenseAcceleration=off  SenseTorqueForce=off  SenseLowerLimitTorqueForce=off  SenseUpperLimitTorqueForce=off
  palm_link11 : Subsystem
  palm_link21 : Subsystem
  palm_link31 : Subsystem
  f3_in1 : PMIOPort  Side=Left
  f3_in2 : PMIOPort  Port=2  Side=Left
  f3_in3 : PMIOPort  Port=3  Side=Left
  f3_in4 : PMIOPort  Port=4  Side=Left
  f2_in1 : PMIOPort  Port=5  Side=Left
  f2_in2 : PMIOPort  Port=6  Side=Left
  f2_in3 : PMIOPort  Port=7  Side=Left
  f2_in4 : PMIOPort  Port=8  Side=Left
  f1_in1 : PMIOPort  Port=9  Side=Left
  f1_in2 : PMIOPort  Port=10  Side=Left
  f1_in3 : PMIOPort  Port=11  Side=Left
  f1_in4 : PMIOPort  Port=12  Side=Left
  f3_out1 : PMIOPort  Port=13  Side=Right
  f3_out2 : PMIOPort  Port=14  Side=Right
  f3_out3 : PMIOPort  Port=15  Side=Right
  f3_out4 : PMIOPort  Port=16  Side=Right
  f2_out1 : PMIOPort  Port=17  Side=Right
  f2_out2 : PMIOPort  Port=18  Side=Right
  f2_out3 : PMIOPort  Port=19  Side=Right
  f2_out4 : PMIOPort  Port=20  Side=Right
  f1_out1 : PMIOPort  Port=21  Side=Right
  f1_out2 : PMIOPort  Port=22  Side=Right
  f1_out3 : PMIOPort  Port=23  Side=Right
  f1_out4 : PMIOPort  Port=24  Side=Right
  connections:
  base_link/LConn1 -- MechanismConfiguration/RConn1 -- Solver Configuration/RConn1 -- World/RConn1
  finger_joint_3_2/RConn1 -- finger_link321/LConn1
  finger_joint_2_2/LConn1 -- finger_link211/RConn1
  palm_joint_1/RConn1 -- palm_link11/LConn1
  palm_joint_2/RConn1 -- palm_link21/LConn1
  finger_joint_3_3/LConn1 -- finger_link321/RConn1
  finger_joint_2_1/RConn1 -- finger_link211/LConn1
  finger_joint_1_3/RConn1 -- finger_link131/LConn1
  finger_joint_2_1/LConn1 -- palm_link21/RConn1
  finger_joint_2_3/RConn1 -- finger_link231/LConn1
  base_link/RConn1 -- palm_joint_3/LConn1
  finger_joint_1_1/LConn1 -- palm_link11/RConn1
  finger_joint_2_2/RConn1 -- finger_link221/LConn1
  finger_joint_1_3/LConn1 -- finger_link121/RConn1
  finger_joint_2_3/LConn1 -- finger_link221/RConn1
  finger_joint_1_2/LConn1 -- finger_link111/RConn1
  base_link/RConn3 -- palm_joint_1/LConn1
  palm_joint_3/RConn1 -- palm_link31/LConn1
  finger_joint_3_1/LConn1 -- palm_link31/RConn1
  finger_joint_3_1/RConn1 -- finger_link311/LConn1
  base_link/RConn2 -- palm_joint_2/LConn1
  finger_joint_3_2/LConn1 -- finger_link311/RConn1
  finger_joint_3_3/RConn1 -- finger_link331/LConn1
  finger_joint_1_2/RConn1 -- finger_link121/LConn1
  finger_joint_1_1/RConn1 -- finger_link111/LConn1
  f3_in1/RConn1 -- palm_joint_3/LConn2
  f3_in2/RConn1 -- finger_joint_3_1/LConn2
  f3_in3/RConn1 -- finger_joint_3_2/LConn2
  f3_in4/RConn1 -- finger_joint_3_3/LConn2
  f3_out1/RConn1 -- palm_joint_3/RConn2
  f3_out2/RConn1 -- finger_joint_3_1/RConn2
  f3_out3/RConn1 -- finger_joint_3_2/RConn2
  f3_out4/RConn1 -- finger_joint_3_3/RConn2
  f2_in1/RConn1 -- palm_joint_2/LConn2
  f2_in2/RConn1 -- finger_joint_2_1/LConn2
  f2_in3/RConn1 -- finger_joint_2_2/LConn2
  f2_in4/RConn1 -- finger_joint_2_3/LConn2
  f1_in1/RConn1 -- palm_joint_1/LConn2
  f1_in2/RConn1 -- finger_joint_1_1/LConn2
  f1_in3/RConn1 -- finger_joint_1_2/LConn2
  f1_in4/RConn1 -- finger_joint_1_3/LConn2
  f2_out1/RConn1 -- palm_joint_2/RConn2
  f2_out2/RConn1 -- finger_joint_2_1/RConn2
  f2_out3/RConn1 -- finger_joint_2_2/RConn2
  f2_out4/RConn1 -- finger_joint_2_3/RConn2
  f1_out1/RConn1 -- palm_joint_1/RConn2
  f1_out2/RConn1 -- finger_joint_1_1/RConn2
  f1_out3/RConn1 -- finger_joint_1_2/RConn2
  f1_out4/RConn1 -- finger_joint_1_3/RConn2

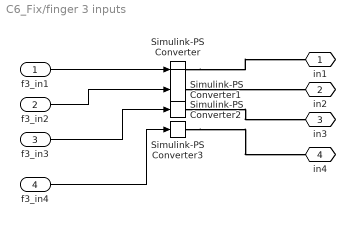
== system C6_Fix/finger 3 inputs ==
  f3_in1 : Inport
  f3_in2 : Inport  Port=2
  f3_in3 : Inport  Port=3
  f3_in4 : Inport  Port=4
  Simulink-PS Converter{,1..3} (4 alike) : nesl_utility/Simulink-PS Converter  PhysicalDomain=network_engine_domain  SubClassName=ps_input  LeftPortType=input  RightPortType=output  PseudoPeriodic=off  Frequencies=[]  NoiseDistribution=none  NoiseParameters=[]  Unit=1  AffineConversion=off  FilteringAndDerivatives=provide  SimscapeFilterOrder=1  InputFilterTimeConstant=0.001  UdotUserProvided=0
  in1 : PMIOPort  Side=Right
  in2 : PMIOPort  Port=2  Side=Right
  in3 : PMIOPort  Port=3  Side=Right
  in4 : PMIOPort  Port=4  Side=Right
  wires:
  f3_in1/1 -> Simulink-PS Converter/1
  f3_in2/1 -> Simulink-PS Converter1/1
  f3_in3/1 -> Simulink-PS Converter2/1
  f3_in4/1 -> Simulink-PS Converter3/1
  connections:
  Simulink-PS Converter/RConn1 -- in1/RConn1
  Simulink-PS Converter3/RConn1 -- in4/RConn1
  Simulink-PS Converter1/RConn1 -- in2/RConn1
  Simulink-PS Converter2/RConn1 -- in3/RConn1

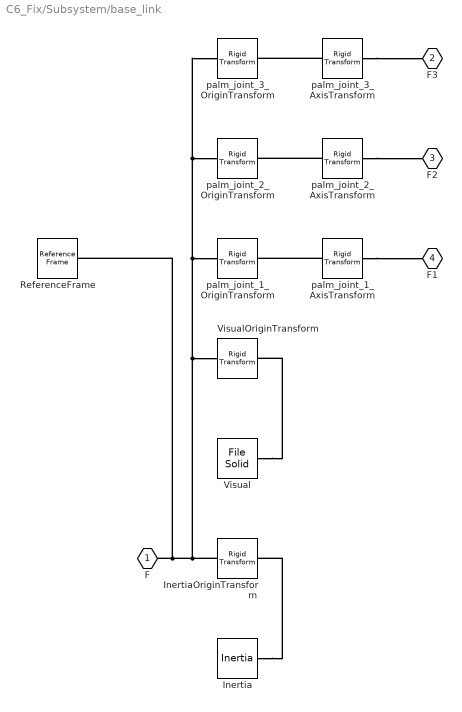
== system C6_Fix/Subsystem/base_link ==
  Inertia : sm_lib/Body Elements/Inertia  InertiaType=Custom  Mass=0.196862396727556  MassUnits=kg  CenterOfMass=[0, 0, 0]  CenterOfMassUnits=m  MomentsOfInertia=[0.000142852426045108, 0.0001428931233289563, 0.0002203151480814937]  MomentsOfInertiaUnits=kg*m^2  ProductsOfInertia=[-5.326694760190293e-14, 4.087505542588535e-09, -1.42337964331718e-13]  ProductsOfInertiaUnits=kg*m^2  GraphicType=None  MarkerShape=Inertia  MarkerSize=20  GraphicVisPropType=SimpleVisualProperties  GraphicDiffuseColor=[0.5 0.5 0.5]  GraphicOpacity=1  GraphicSpecularColor=[0.5 0.5 0.5 1.0]  GraphicAmbientColor=[0.15 0.15 0.15 1.0]  GraphicEmissiveColor=[0.0 0.0 0.0 1.0]  GraphicShininess=75
  InertiaOriginTransform : sm_lib/Frames and Transforms/Rigid Transform  RotationMethod=RotationSequence  FollAlignAxisA=+X  BaseAlignAxisA=+Y  FollAlignAxisB=+Y  BaseAlignAxisB=+Z  RotationStandardAxis=+Z  RotationAngle=0  RotationAngleUnits=deg  RotationArbitraryAxis=[0 0 1]  RotationSequenceAxes=BaseAxes  RotationSequence=XYZ  RotationSequenceAngles=[0, 0, 0]  RotationSequenceAnglesUnits=rad  RotationMatrix=[1 0 0;0 1 0;0 0 1]  Quaternion=[1 0 0 0]  TranslationMethod=Cartesian  TranslationCartesianOffset=[0.2824084412039216, -0.01747868073746133, -0.008955658350251127]  TranslationCartesianOffsetUnits=m  TranslationStandardAxis=+Z  TranslationStandardOffset=0  TranslationStandardOffsetUnits=m  TranslationROffset=0  TranslationROffsetUnits=m  TranslationThetaOffset=0  TranslationThetaOffsetUnits=deg  TranslationZOffset=0  TranslationZOffsetUnits=m
  ReferenceFrame : sm_lib/Frames and Transforms/Reference Frame
  Visual : sm_lib/Body Elements/File Solid  ExtGeomFileName=C:\Users\steph\OneDrive\Desktop\URDF_C6_Fix\Space_Gripper_URDF_fix\meshes\base_link.stl  UnitType=Custom  ExtGeomFileUnits=mm  StepReaderType=HEX  ExportConvexHullGeometry=off  InertiaType=Custom  BasedOnType=DensityFromFile  Density=1000  DensityUnits=kg/m^3  Mass=0  MassUnits=kg  CenterOfMass=[0, 0, 0]  CenterOfMassUnits=m  MomentsOfInertia=[0, 0, 0]  MomentsOfInertiaUnits=kg*m^2  ProductsOfInertia=[0, 0, 0]  ProductsOfInertiaUnits=kg*m^2  GraphicType=FromGeometry  MarkerShape=Sphere  MarkerSize=10  GraphicVisPropType=SimpleVisualProperties  GraphicDiffuseColor=[0.6353 0.07843 0.1843]  GraphicOpacity=1  GraphicSpecularColor=[0.5 0.5 0.5 1.0]  GraphicAmbientColor=[0.15 0.15 0.15 1.0]  GraphicEmissiveColor=[0.0 0.0 0.0 1.0]  GraphicShininess=75  DoExposeReferenceFrame=on  SerializedFrames=<Frames/>
  VisualOriginTransform : sm_lib/Frames and Transforms/Rigid Transform  RotationMethod=RotationSequence  FollAlignAxisA=+X  BaseAlignAxisA=+Y  FollAlignAxisB=+Y  BaseAlignAxisB=+Z  RotationStandardAxis=+Z  RotationAngle=0  RotationAngleUnits=deg  RotationArbitraryAxis=[0 0 1]  RotationSequenceAxes=BaseAxes  RotationSequence=XYZ  RotationSequenceAngles=[0, 0, 0]  RotationSequenceAnglesUnits=rad  RotationMatrix=[1 0 0;0 1 0;0 0 1]  Quaternion=[1 0 0 0]  TranslationMethod=Cartesian  TranslationCartesianOffset=[0, 0, 0]  TranslationCartesianOffsetUnits=m  TranslationStandardAxis=+Z  TranslationStandardOffset=0  TranslationStandardOffsetUnits=m  TranslationROffset=0  TranslationROffsetUnits=m  TranslationThetaOffset=0  TranslationThetaOffsetUnits=deg  TranslationZOffset=0  TranslationZOffsetUnits=m
  palm_joint_1_AxisTransform : sm_lib/Frames and Transforms/Rigid Transform  RotationMethod=ArbitraryAxis  FollAlignAxisA=+X  BaseAlignAxisA=+Y  FollAlignAxisB=+Y  BaseAlignAxisB=+Z  RotationStandardAxis=+Z  RotationAngle=0  RotationAngleUnits=rad  RotationArbitraryAxis=[1, 0, 0]  RotationSequenceAxes=FollowerAxes  RotationSequence=XYX  RotationSequenceAngles=[0 0 0]  RotationSequenceAnglesUnits=deg  RotationMatrix=[1 0 0;0 1 0;0 0 1]  Quaternion=[1 0 0 0]  TranslationMethod=Cartesian  TranslationCartesianOffset=[0, 0, 0]  TranslationCartesianOffsetUnits=m  TranslationStandardAxis=+Z  TranslationStandardOffset=0  TranslationStandardOffsetUnits=m  TranslationROffset=0  TranslationROffsetUnits=m  TranslationThetaOffset=0  TranslationThetaOffsetUnits=deg  TranslationZOffset=0  TranslationZOffsetUnits=m
  palm_joint_1_OriginTransform : sm_lib/Frames and Transforms/Rigid Transform  RotationMethod=RotationSequence  FollAlignAxisA=+X  BaseAlignAxisA=+Y  FollAlignAxisB=+Y  BaseAlignAxisB=+Z  RotationStandardAxis=+Z  RotationAngle=0  RotationAngleUnits=deg  RotationArbitraryAxis=[0 0 1]  RotationSequenceAxes=BaseAxes  RotationSequence=XYZ  RotationSequenceAngles=[0, 0, 0]  RotationSequenceAnglesUnits=rad  RotationMatrix=[1 0 0;0 1 0;0 0 1]  Quaternion=[1 0 0 0]  TranslationMethod=Cartesian  TranslationCartesianOffset=[0.252173, -0.016479, -0.010014]  TranslationCartesianOffsetUnits=m  TranslationStandardAxis=+Z  TranslationStandardOffset=0  TranslationStandardOffsetUnits=m  TranslationROffset=0  TranslationROffsetUnits=m  TranslationThetaOffset=0  TranslationThetaOffsetUnits=deg  TranslationZOffset=0  TranslationZOffsetUnits=m
  palm_joint_2_AxisTransform : sm_lib/Frames and Transforms/Rigid Transform  RotationMethod=ArbitraryAxis  FollAlignAxisA=+X  BaseAlignAxisA=+Y  FollAlignAxisB=+Y  BaseAlignAxisB=+Z  RotationStandardAxis=+Z  RotationAngle=0  RotationAngleUnits=rad  RotationArbitraryAxis=[1, 0, 0]  RotationSequenceAxes=FollowerAxes  RotationSequence=XYX  RotationSequenceAngles=[0 0 0]  RotationSequenceAnglesUnits=deg  RotationMatrix=[1 0 0;0 1 0;0 0 1]  Quaternion=[1 0 0 0]  TranslationMethod=Cartesian  TranslationCartesianOffset=[0, 0, 0]  TranslationCartesianOffsetUnits=m  TranslationStandardAxis=+Z  TranslationStandardOffset=0  TranslationStandardOffsetUnits=m  TranslationROffset=0  TranslationROffsetUnits=m  TranslationThetaOffset=0  TranslationThetaOffsetUnits=deg  TranslationZOffset=0  TranslationZOffsetUnits=m
  palm_joint_2_OriginTransform : sm_lib/Frames and Transforms/Rigid Transform  RotationMethod=RotationSequence  FollAlignAxisA=+X  BaseAlignAxisA=+Y  FollAlignAxisB=+Y  BaseAlignAxisB=+Z  RotationStandardAxis=+Z  RotationAngle=0  RotationAngleUnits=deg  RotationArbitraryAxis=[0 0 1]  RotationSequenceAxes=BaseAxes  RotationSequence=XYZ  RotationSequenceAngles=[0, 0, 0]  RotationSequenceAnglesUnits=rad  RotationMatrix=[1 0 0;0 1 0;0 0 1]  Quaternion=[1 0 0 0]  TranslationMethod=Cartesian  TranslationCartesianOffset=[0.296629, -0.044146, -0.010014]  TranslationCartesianOffsetUnits=m  TranslationStandardAxis=+Z  TranslationStandardOffset=0  TranslationStandardOffsetUnits=m  TranslationROffset=0  TranslationROffsetUnits=m  TranslationThetaOffset=0  TranslationThetaOffsetUnits=deg  TranslationZOffset=0  TranslationZOffsetUnits=m
  palm_joint_3_AxisTransform : sm_lib/Frames and Transforms/Rigid Transform  RotationMethod=ArbitraryAxis  FollAlignAxisA=+X  BaseAlignAxisA=+Y  FollAlignAxisB=+Y  BaseAlignAxisB=+Z  RotationStandardAxis=+Z  RotationAngle=0  RotationAngleUnits=rad  RotationArbitraryAxis=[1, 0, 0]  RotationSequenceAxes=FollowerAxes  RotationSequence=XYX  RotationSequenceAngles=[0 0 0]  RotationSequenceAnglesUnits=deg  RotationMatrix=[1 0 0;0 1 0;0 0 1]  Quaternion=[1 0 0 0]  TranslationMethod=Cartesian  TranslationCartesianOffset=[0, 0, 0]  TranslationCartesianOffsetUnits=m  TranslationStandardAxis=+Z  TranslationStandardOffset=0  TranslationStandardOffsetUnits=m  TranslationROffset=0  TranslationROffsetUnits=m  TranslationThetaOffset=0  TranslationThetaOffsetUnits=deg  TranslationZOffset=0  TranslationZOffsetUnits=m
  palm_joint_3_OriginTransform : sm_lib/Frames and Transforms/Rigid Transform  RotationMethod=RotationSequence  FollAlignAxisA=+X  BaseAlignAxisA=+Y  FollAlignAxisB=+Y  BaseAlignAxisB=+Z  RotationStandardAxis=+Z  RotationAngle=0  RotationAngleUnits=deg  RotationArbitraryAxis=[0 0 1]  RotationSequenceAxes=BaseAxes  RotationSequence=XYZ  RotationSequenceAngles=[0, 0, 0]  RotationSequenceAnglesUnits=rad  RotationMatrix=[1 0 0;0 1 0;0 0 1]  Quaternion=[1 0 0 0]  TranslationMethod=Cartesian  TranslationCartesianOffset=[0.298361, 0.008188000000000001, -0.010014]  TranslationCartesianOffsetUnits=m  TranslationStandardAxis=+Z  TranslationStandardOffset=0  TranslationStandardOffsetUnits=m  TranslationROffset=0  TranslationROffsetUnits=m  TranslationThetaOffset=0  TranslationThetaOffsetUnits=deg  TranslationZOffset=0  TranslationZOffsetUnits=m
  F : PMIOPort  Side=Left
  F3 : PMIOPort  Port=2  Side=Right
  F2 : PMIOPort  Port=3  Side=Right
  F1 : PMIOPort  Port=4  Side=Right
  connections:
  Inertia/RConn1 -- InertiaOriginTransform/RConn1
  InertiaOriginTransform/LConn1 -- ReferenceFrame/RConn1 -- F/RConn1 -- palm_joint_2_OriginTransform/LConn1 -- palm_joint_3_OriginTransform/LConn1 -- palm_joint_1_OriginTransform/LConn1 -- VisualOriginTransform/LConn1
  Visual/RConn1 -- VisualOriginTransform/RConn1
  palm_joint_1_AxisTransform/RConn1 -- F1/RConn1
  palm_joint_1_AxisTransform/LConn1 -- palm_joint_1_OriginTransform/RConn1
  palm_joint_2_AxisTransform/RConn1 -- F2/RConn1
  palm_joint_2_AxisTransform/LConn1 -- palm_joint_2_OriginTransform/RConn1
  palm_joint_3_AxisTransform/RConn1 -- F3/RConn1
  palm_joint_3_AxisTransform/LConn1 -- palm_joint_3_OriginTransform/RConn1
